simulink model "msingleinst"  (Simulink 8.0)
settings: Solver=FixedStepDiscrete  SolverMode=SingleTasking  StartTime=0.0  StopTime=10.0  RelTol=1e-3
undefined symbols (not defined in the file or in its folder): i
settings Model: FPTRunName=Active  Creator=mani  LastModifiedBy=yshang  ExtModeAutoUpdateStatusClock=off
settings DataIOCC: SaveFormat=StructureWithTime  SignalLoggingSaveFormat=ModelDataLogs  SignalLoggingName=sigsOut
settings OptimizationCC: InlineParams=on  InlineInvariantSignals=on  InitFltsAndDblsToZero=on  BufferReusableBoundary=off
settings DebuggingCC: SaveWithParameterizedLinksMsg=none  SignalResolutionControl=TryResolveAllWithWarning  SolverPrmCheckMsg=none  MultiTaskDSMMsg=warning  MultiTaskCondExecSysMsg=none  SigSpecEnsureSampleTimeMsg=none  FcnCallInpInsideContextMsg=Use local settings
settings HardwareCC: TargetUnknown=on
settings RTWCC: IncludeERTFirstTime=on
settings GRTTargetCC: TargetFcnLib=ansi_tfl_tmw.mat  CombineOutputUpdateFcns=off

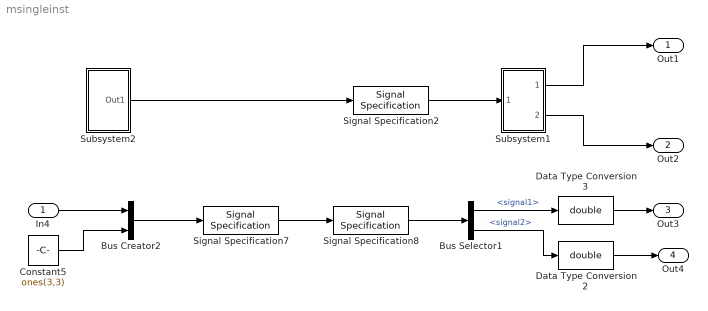
== system msingleinst ==
  In4 : Inport  OutDataTypeStr=fixdt(0,16,10)  PortDimensions=[2,5]  SampleTime=5
      settings: SignalType=complex
  Bus Creator2 : BusCreator  Inputs=2
  Bus Selector1 : BusSelector  OutputSignals=signal1,signal2
  Constant5 : Constant  Value=ones(3,3)  OutDataTypeStr=double  SampleTime=0.5
  Data Type Conversion2 : DataTypeConversion  OutDataTypeStr=double  SaturateOnIntegerOverflow=on  RndMeth=Zero
  Data Type Conversion3 : DataTypeConversion  OutDataTypeStr=double  SaturateOnIntegerOverflow=on  RndMeth=Zero
  Signal Specification2 : SignalSpecification
  Signal Specification7 : SignalSpecification
  Signal Specification8 : SignalSpecification
  Subsystem1 : Subsystem  TreatAsAtomicUnit=on
  Subsystem2 : Subsystem  TreatAsAtomicUnit=on
  Out1 : Outport
  Out2 : Outport  Port=2
  Out3 : Outport  Port=3
  Out4 : Outport  Port=4
  wires:
  Subsystem2/1(Out1) -> Signal Specification2/1
  Signal Specification2/1 -> Subsystem1/1(In1)
  Bus Creator2/1 -> Signal Specification7/1
  In4/1 -> Bus Creator2/1
  Constant5/1 -> Bus Creator2/2
  Bus Selector1/1 -> Data Type Conversion3/1  "<signal1>"
  Bus Selector1/2 -> Data Type Conversion2/1  "<signal2>"
  Data Type Conversion2/1 -> Out4/1
  Data Type Conversion3/1 -> Out3/1
  Signal Specification7/1 -> Signal Specification8/1
  Signal Specification8/1 -> Bus Selector1/1
  Subsystem1/1(Out3) -> Out1/1
  Subsystem1/2(Out4) -> Out2/1

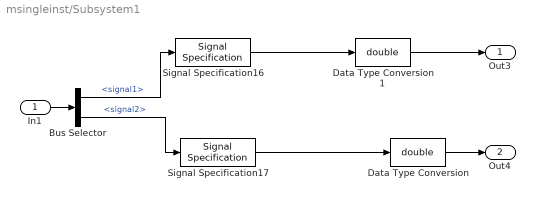
== system msingleinst/Subsystem1 ==
  In1 : Inport
  Bus Selector : BusSelector  OutputSignals=signal1,signal2
  Data Type Conversion : DataTypeConversion  OutDataTypeStr=double  SaturateOnIntegerOverflow=on  RndMeth=Zero
  Data Type Conversion1 : DataTypeConversion  OutDataTypeStr=double  SaturateOnIntegerOverflow=on  RndMeth=Zero
  Signal Specification16 : SignalSpecification  OutDataTypeStr=fixdt(1,16,10)  Dimensions=[2,2]  SampleTime=1.0
      settings: SignalType=complex
  Signal Specification17 : SignalSpecification  OutDataTypeStr=boolean  Dimensions=[3,3]  SampleTime=5
      settings: SignalType=complex
  Out3 : Outport
  Out4 : Outport  Port=2
  wires:
  Bus Selector/1 -> Signal Specification16/1  "<signal1>"
  Bus Selector/2 -> Signal Specification17/1  "<signal2>"
  Data Type Conversion/1 -> Out4/1
  Data Type Conversion1/1 -> Out3/1
  Signal Specification16/1 -> Data Type Conversion1/1
  Signal Specification17/1 -> Data Type Conversion/1
  In1/1 -> Bus Selector/1

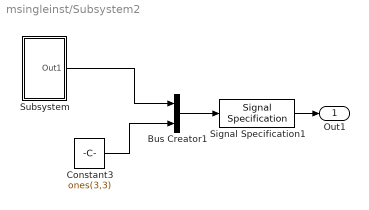
== system msingleinst/Subsystem2 ==
  Bus Creator1 : BusCreator  Inputs=2
  Constant3 : Constant  Value=ones(3,3)  OutDataTypeStr=Inherit: Inherit via back propagation
  Signal Specification1 : SignalSpecification
  Subsystem : Subsystem  TreatAsAtomicUnit=on
      settings: RTWSystemCode=Function
  Out1 : Outport
  wires:
  Bus Creator1/1 -> Signal Specification1/1
  Subsystem/1(Out1) -> Bus Creator1/1
  Constant3/1 -> Bus Creator1/2
  Signal Specification1/1 -> Out1/1

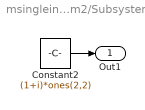
== system msingleinst/Subsystem2/Subsystem ==
  Constant2 : Constant  Value=(1+i)*ones(2,2)  OutDataTypeStr=Inherit: Inherit via back propagation
  Out1 : Outport
  wires:
  Constant2/1 -> Out1/1
